simulink model "P3p3"  (R2017a)
settings: Solver=ode1  StartTime=0.0  StopTime=inf  FixedStep=0.01  RelTol=1e-3  EnableMultiTasking=on
PostLoadFcn:
  | qc_set_target_type(getConfigSet(bdroot, 'QUARC Default Target Configuration'));
values from neighbouring files (symbols this model uses):
  Joystick_gain_x = 1    [P3p3_init.m]
  Joystick_gain_y = -1    [P3p3_init.m]
  K = lqr(A_PI, B_PI, Q, R)    [P3p3_init.m]
  l_2 = g*(l_c*m_c - 2*m_p * l_h)    (= -0.659232)    [P3p3_init.m]
  l_3 = l_h * k_f    (= 0.10464)    [P3p3_init.m]
  P = inv(C_P*inv(B_P*K(:,1:3) - A_P) * B_P)    [P3p3_init.m]
undefined symbols (not defined in the file or in its folder): HIL, qc_get_step_size
libraries: simulink_extras x6, quarc_library x4
settings Model: SimulationMode=external  ExtModeTrigDuration=5000  Creator=Rchan  LastModifiedBy=Jakob
settings SolverCC: PositivePriorityOrder=on
settings DataIOCC: LimitDataPoints=on  SaveFormat=Array  SignalLoggingSaveFormat=ModelDataLogs
settings OptimizationCC: ExpressionDepthLimit=2147483647  InitFltsAndDblsToZero=on  LifeSpan=inf
settings DebuggingCC: SaveWithParameterizedLinksMsg=none  UnderspecifiedInitializationDetection=Classic  MergeDetectMultiDrivingBlocksExec=none  SolverPrmCheckMsg=warning  MultiTaskDSMMsg=warning  MultiTaskCondExecSysMsg=none  FcnCallInpInsideContextMsg=warning  StateNameClashWarn=warning  SFUnexpectedBacktrackingDiag=warning  SFNoUnconditionalDefaultTransitionDiag=warning  SFExecutionAtInitializationDiag=none
settings HardwareCC: ProdBitPerPointer=32  ProdBitPerSizeT=32  ProdBitPerPtrDiffT=32  ProdLargestAtomicFloat=None  ProdIntDivRoundTo=Undefined  ProdEndianess=Unspecified  ProdWordSize=32  ProdHWDeviceType=32-bit Generic
settings ModelReferenceCC: PropagateSignalLabelsOutOfModel=off
settings RTWCC: SystemTargetFile=quarc_win64.tlc  TemplateMakefile=quarc_default_tmf  Description=QUARC Win64 Target
settings STFCustomTargetCC: TargetPreCompLibLocation=C:\PROGRA~3\QUARC\lib\2014a\win64\release  ConcurrentExecutionCompliant=on  GeneratePreprocessorConditionals=Disable all  CPPClassGenCompliant=on  SystemTargetFile=quarc_win64.tlc
settings GRTTargetCC: TargetPreCompLibLocation=C:\PROGRA~3\QUARC\lib\2014a\win64\release  TargetLangStandard=C89/C90 (ANSI)  ParMdlRefBuildCompliant=off  CompOptLevelCompliant=off  GeneratePreprocessorConditionals=Disable all  CombineOutputUpdateFcns=off  MatFileLogging=off  GRTInterface=on  UseToolchainInfoCompliant=off  ExtMode=on  ExtModeMexFile=quarc_comm
settings ConfigComp: CovMetricSettings=dw  CovHtmlReporting=on  CovSaveCumulativeToWorkspaceVar=on  CovSaveSingleToWorkspaceVar=on  CovExternalEMLEnable=off  CovSFcnEnable=off

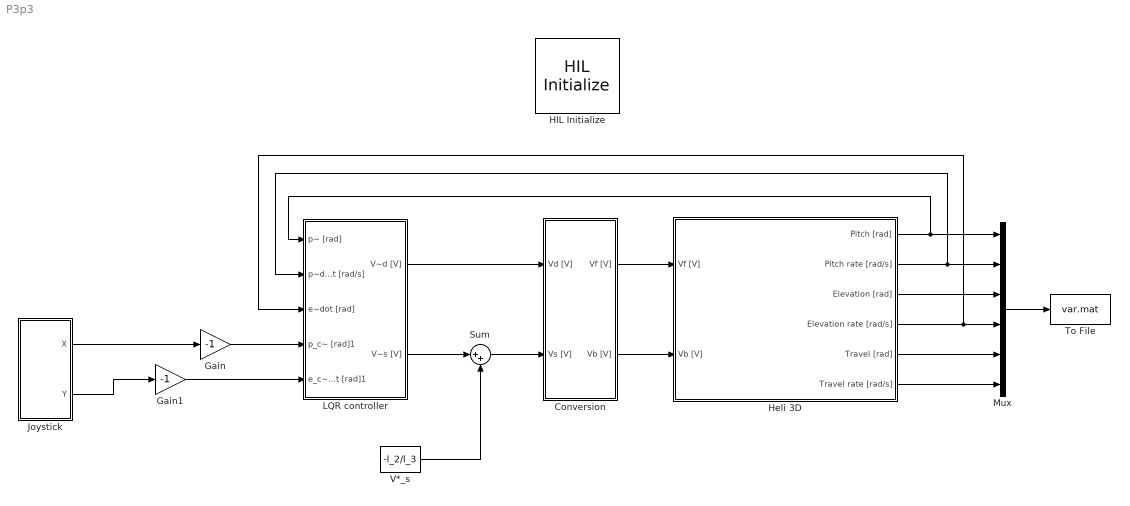
== system P3p3 ==
  Conversion : Subsystem
  Gain : Gain  Gain=-1
  Gain1 : Gain  Gain=-1
  HIL Initialize : quarc_library/Data Acquisition/Generic/Configuration/HIL Initialize  Priority=-99  object_name=HIL-1  board_type=q8_usb  board_number=0  board_options=update_rate=normal;decimation=1  exclusive=off  active=off  hardware_clocks=[0:2]  clock_modes=[]  initial_clock_frequencies=[]  set_clock_params_at_start=off  set_clock_params_at_switch_in=off  set_clock_frequencies_at_start=off  set_clock_frequencies_at_switch_in=off  analog_input_channels=[0:7]  analog_input_maximums=10  analog_input_minimums=-10  set_analog_input_params_at_start=on  set_analog_input_params_at_switch_in=off  analog_output_channels=[0:7]  analog_output_maximums=10  analog_output_minimums=-10  initial_analog_outputs=[0]  final_analog_outputs=[0]  watchdog_analog_outputs=0  set_analog_output_params_at_start=on  set_analog_output_params_at_switch_in=off  set_analog_outputs_at_start=on  set_analog_outputs_at_switch_in=off  set_analog_outputs_at_terminate=on  set_analog_outputs_at_switch_out=off  set_analog_outputs_on_watchdog=off  digital_input_channels=[]  digital_output_channels=[]  digital_output_configuration=[]  initial_digital_outputs=[1]  final_digital_outputs=[1]  watchdog_digital_outputs=[1]  set_digital_output_params_at_start=off  set_digital_output_params_at_switch_in=off  set_digital_outputs_at_start=on  set_digital_outputs_at_switch_in=off  set_digital_outputs_at_terminate=on  set_digital_outputs_at_switch_out=off  set_digital_outputs_on_watchdog=off  encoder_channels=[0:7]  quadrature=[4]  encoder_filter_frequency=[]  initial_encoder_counts=[0]  set_encoder_params_at_start=on  set_encoder_params_at_switch_in=off  set_encoder_counts_at_start=on  set_encoder_counts_at_switch_in=off  pwm_channels=[0:7]  pwm_modes=0  pwm_frequency=99.532799999999995e6/4095  pwm_configuration=[0]  pwm_alignment=[0]  pwm_polarity=[1]  pwm_leading_deadband=[0]  pwm_trailing_deadband=[0]  initial_pwm_outputs=[0]  final_pwm_outputs=[0]  watchdog_pwm_outputs=[0]  set_pwm_params_at_start=on  set_pwm_params_at_switch_in=off  set_pwm_outputs_at_start=on  set_pwm_outputs_at_switch_in=off  set_pwm_outputs_at_terminate=on  set_pwm_outputs_at_switch_out=off  set_pwm_outputs_on_watchdog=off  other_output_channels=[]  initial_other_outputs=[]  final_other_outputs=[]  watchdog_other_outputs=[]  set_other_outputs_at_start=off  set_other_outputs_at_switch_in=off  set_other_outputs_at_terminate=off  set_other_outputs_at_switch_out=off  set_other_outputs_on_watchdog=off
  Heli 3D : Subsystem
  Joystick : Subsystem
  LQR controller : Subsystem
  Mux : Mux  Inputs=6
  Sum : Sum  Inputs=|++
  To File : ToFile  Filename=var.mat  MatrixName=var
  V*_s : Constant  Value=-l_2/l_3
  wires:
  Conversion/2(Vb [V]) -> Heli 3D/2(Vb [V])
  Conversion/1(Vf [V]) -> Heli 3D/1(Vf [V])
  Heli 3D/5(Travel [rad]) -> Mux/5
  Heli 3D/6(Travel rate [rad/s]) -> Mux/6
  Heli 3D/1(Pitch [rad]) -> Mux/1, LQR controller/1(p~ [rad])
  Heli 3D/2(Pitch rate [rad/s]) -> Mux/2, LQR controller/2(p~dot [rad/s])
  Mux/1 -> To File/1
  Heli 3D/4(Elevation rate [rad/s]) -> LQR controller/3(e~dot [rad]), Mux/4
  Heli 3D/3(Elevation [rad]) -> Mux/3
  Joystick/1(X) -> Gain/1
  LQR controller/1("V~d [V] ") -> Conversion/1(Vd [V])
  Gain1/1 -> LQR controller/5(e_c~dot [rad]1)
  Gain/1 -> LQR controller/4(p_c~ [rad]1)
  Joystick/2(Y) -> Gain1/1
  V*_s/1 -> Sum/2
  Sum/1 -> Conversion/2(Vs [V])
  LQR controller/2(V~s [V]) -> Sum/1

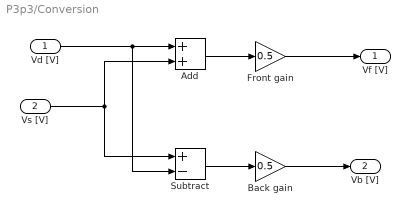
== system P3p3/Conversion ==
  Vd [V] : Inport
  Vs [V] : Inport  Port=2
  Add : Sum
  Back gain : Gain  Gain=0.5
  Front gain : Gain  Gain=0.5
  Subtract : Sum  Inputs=+-
  Vf [V] : Outport
  Vb [V] : Outport  Port=2
  wires:
  Vd [V]/1 -> Subtract/2, Add/1
  Vs [V]/1 -> Subtract/1, Add/2
  Subtract/1 -> Back gain/1
  Back gain/1 -> Vb [V]/1
  Add/1 -> Front gain/1
  Front gain/1 -> Vf [V]/1

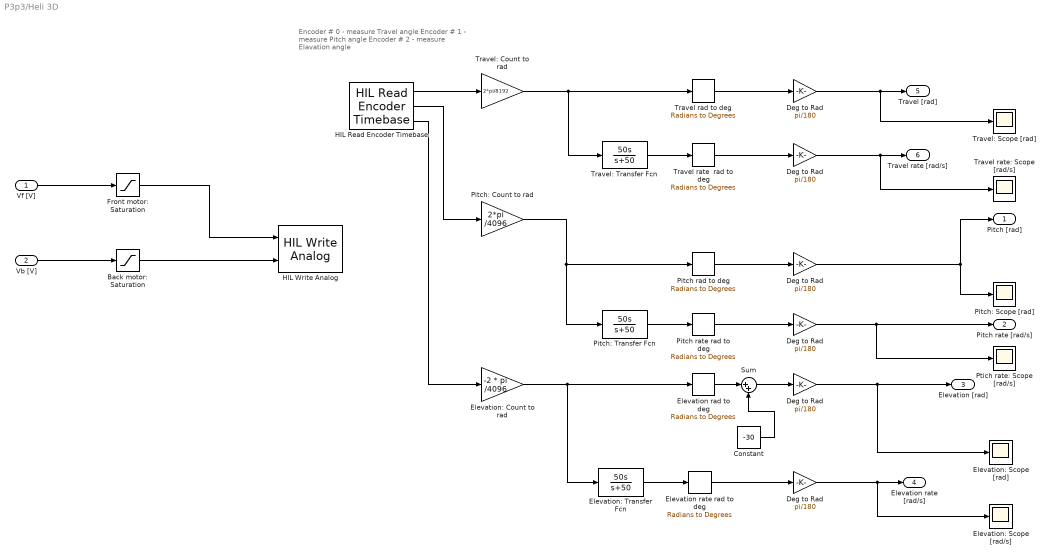
== system P3p3/Heli 3D ==
  note: Encoder # 0 - measure Travel angle
      | Encoder # 1 - measure Pitch angle
      | Encoder # 2 - measure Elavation angle
  Vf [V] : Inport
  Vb [V] : Inport  Port=2
  Back motor: Saturation : Saturate  UpperLimit=5  LowerLimit=-5
  Constant : Constant  Value=-30
  Deg to Rad : Gain  Gain=pi/180
  "Deg to Rad  " : Gain  Gain=pi/180
  "Deg to Rad   " : Gain  Gain=pi/180
  "Deg to Rad    " : Gain  Gain=pi/180
  "Deg to Rad     " : Gain  Gain=pi/180
  "Deg to Rad      " : Gain  Gain=pi/180
  Elevation rad to deg : simulink_extras/Transformations/Radians to Degrees
  Elevation rate rad to deg : simulink_extras/Transformations/Radians to Degrees
  Elevation: Count to rad : Gain  Gain=-2 * pi /4096
  Elevation: Scope [rad/s] : Scope
  Elevation: Scope [rad] : Scope
  Elevation: Transfer Fcn : TransferFcn  Numerator=[50 0]  Denominator=[1 50]
  Front motor: Saturation : Saturate  UpperLimit=5  LowerLimit=-5
  HIL Read Encoder Timebase : quarc_library/Data Acquisition/Generic/Timebases/HIL Read Encoder Timebase  object_name=HIL-1  clock=0  channels=[0:2]  samples_in_buffer=max(ceil(1/qc_get_step_size), 1)  active=on  vector_output=off  data_type_mode=Inherit via back propagation  data_type=double
  HIL Write Analog : quarc_library/Data Acquisition/Generic/Immediate I//O/HIL Write Analog  object_name=HIL-1  channels=[0:1]  sample_time=-1  active=off  vector_input=off
  Pitch rad to deg : simulink_extras/Transformations/Radians to Degrees
  Pitch rate rad to deg : simulink_extras/Transformations/Radians to Degrees
  Pitch: Count to rad : Gain  Gain=2*pi /4096
  Pitch: Scope [rad] : Scope
  Pitch: Transfer Fcn : TransferFcn  Numerator=[50 0]  Denominator=[1 50]
  Ptich rate: Scope [rad/s] : Scope
  Sum : Sum  Inputs=|++
  Travel rad to deg : simulink_extras/Transformations/Radians to Degrees
  Travel rate  rad to deg : simulink_extras/Transformations/Radians to Degrees
  Travel rate: Scope [rad/s] : Scope
  Travel: Count to rad : Gain  Gain=2*pi/8192
  Travel: Scope [rad] : Scope
  Travel: Transfer Fcn : TransferFcn  Numerator=[50 0]  Denominator=[1 50]
  Pitch [rad] : Outport
  Pitch rate [rad/s] : Outport  Port=2
  Elevation [rad] : Outport  Port=3
  Elevation rate [rad/s] : Outport  Port=4
  Travel [rad] : Outport  Port=5
  Travel rate [rad/s] : Outport  Port=6
  wires:
  HIL Read Encoder Timebase/1 -> Travel: Count to rad/1
  HIL Read Encoder Timebase/2 -> Pitch: Count to rad/1
  HIL Read Encoder Timebase/3 -> Elevation: Count to rad/1
  Travel: Count to rad/1 -> Travel: Transfer Fcn/1, Travel rad to deg/1
  Travel: Transfer Fcn/1 -> Travel rate  rad to deg/1
  Pitch: Count to rad/1 -> Pitch: Transfer Fcn/1, Pitch rad to deg/1
  Pitch: Transfer Fcn/1 -> Pitch rate rad to deg/1
  Elevation: Count to rad/1 -> Elevation: Transfer Fcn/1, Elevation rad to deg/1
  Elevation: Transfer Fcn/1 -> Elevation rate rad to deg/1
  Travel rad to deg/1 -> Deg to Rad/1
  Travel rate  rad to deg/1 -> "Deg to Rad  "/1
  Pitch rate rad to deg/1 -> "Deg to Rad    "/1
  Elevation rate rad to deg/1 -> "Deg to Rad      "/1
  Vf [V]/1 -> Front motor: Saturation/1
  Vb [V]/1 -> Back motor: Saturation/1
  Front motor: Saturation/1 -> HIL Write Analog/1
  Back motor: Saturation/1 -> HIL Write Analog/2
  Pitch rad to deg/1 -> "Deg to Rad   "/1
  Constant/1 -> Sum/2
  Sum/1 -> "Deg to Rad     "/1
  Elevation rad to deg/1 -> Sum/1
  "Deg to Rad  "/1 -> Travel rate: Scope [rad/s]/1, Travel rate [rad/s]/1
  Deg to Rad/1 -> Travel: Scope [rad]/1, Travel [rad]/1
  "Deg to Rad   "/1 -> Pitch [rad]/1, Pitch: Scope [rad]/1
  "Deg to Rad    "/1 -> Ptich rate: Scope [rad/s]/1, Pitch rate [rad/s]/1
  "Deg to Rad     "/1 -> Elevation: Scope [rad]/1, Elevation [rad]/1
  "Deg to Rad      "/1 -> Elevation: Scope [rad/s]/1, Elevation rate [rad/s]/1

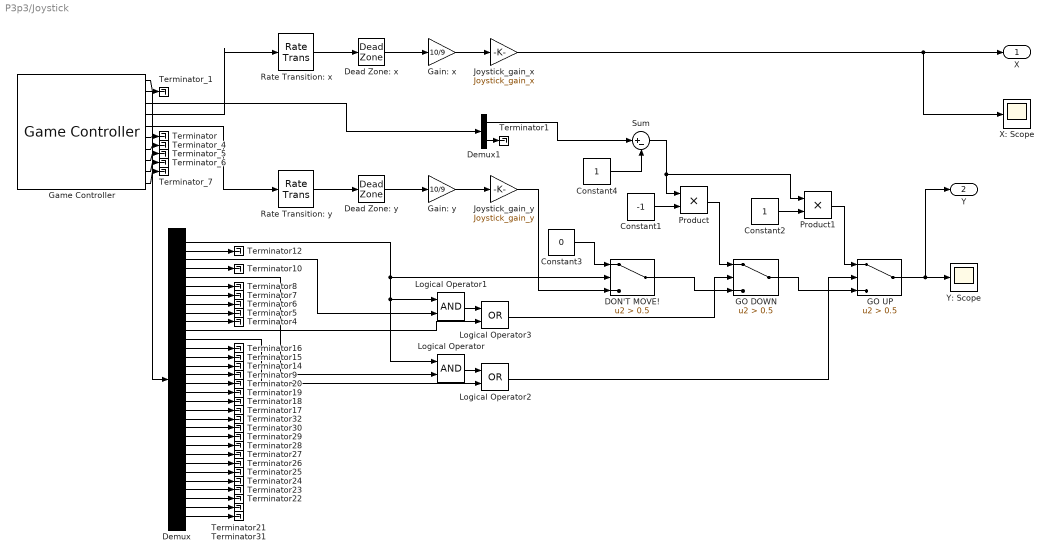
== system P3p3/Joystick ==
  Constant1 : Constant  Value=-1  SampleTime=-1
  Constant2 : Constant  SampleTime=-1
  Constant3 : Constant  Value=0  SampleTime=-1
  Constant4 : Constant  SampleTime=-1
  DON'T MOVE! : Switch  Criteria=u2 > Threshold  Threshold=0.5
  Dead Zone: x : DeadZone  LowerValue=-0.1  UpperValue=0.1  SaturateOnIntegerOverflow=on
  Dead Zone: y : DeadZone  LowerValue=-0.1  UpperValue=0.1  SaturateOnIntegerOverflow=on
  Demux : Demux  Outputs=32
  Demux1 : Demux  Outputs=2
  GO DOWN : Switch  Criteria=u2 > Threshold  Threshold=0.5
  GO UP : Switch  Criteria=u2 > Threshold  Threshold=0.5
  Gain: x : Gain  Gain=10/9
  Gain: y : Gain  Gain=10/9
  Game Controller : quarc_library/Devices/Peripherals/Target/Game Controller  controller=1  buffer_size=12  deadzone=[]  saturation=[]  sample_time=max(qc_get_step_size, 0.01)  auto_center=off  enabled=on
  Joystick_gain_x : Gain  Gain=Joystick_gain_x
  Joystick_gain_y : Gain  Gain=Joystick_gain_y
  Logical Operator : Logic  AllPortsSameDT=off  OutDataTypeStr=boolean
  Logical Operator1 : Logic  AllPortsSameDT=off  OutDataTypeStr=boolean
  Logical Operator2 : Logic  Operator=OR  AllPortsSameDT=off  OutDataTypeStr=boolean
  Logical Operator3 : Logic  Operator=OR  AllPortsSameDT=off  OutDataTypeStr=boolean
  Product : Product
  Product1 : Product
  Rate Transition: x : RateTransition
  Rate Transition: y : RateTransition
  Sum : Sum  Inputs=|+-
  Terminator{,1,4..10,12,14..32} (29 alike) : Terminator
  Terminator_{1,4..7} (5 alike) : Terminator
  X: Scope : Scope
  Y: Scope : Scope
  X : Outport
  Y : Outport  Port=2
  wires:
  Rate Transition: y/1 -> Dead Zone: y/1
  Rate Transition: x/1 -> Dead Zone: x/1
  Game Controller/5 -> Rate Transition: y/1
  Game Controller/4 -> Rate Transition: x/1
  Game Controller/1 -> Terminator_1/1
  Game Controller/7 -> Terminator_4/1
  Game Controller/8 -> Terminator_5/1
  Game Controller/9 -> Terminator_6/1
  Game Controller/10 -> Terminator_7/1
  Game Controller/3 -> Demux1/1
  Game Controller/6 -> Terminator/1
  Dead Zone: x/1 -> Gain: x/1
  Dead Zone: y/1 -> Gain: y/1
  Gain: x/1 -> Joystick_gain_x/1
  Gain: y/1 -> Joystick_gain_y/1
  Game Controller/2 -> Demux/1
  Demux/2 -> Terminator12/1
  Demux/4 -> Terminator10/1
  Demux/7 -> Terminator7/1
  Demux/8 -> Terminator6/1
  Demux/9 -> Terminator5/1
  Demux/10 -> Terminator4/1
  Demux/11 -> Logical Operator3/2
  Demux/12 -> Logical Operator2/2
  Demux/14 -> Terminator15/1
  Demux/15 -> Terminator14/1
  Demux/16 -> Terminator9/1
  Demux/13 -> Terminator16/1
  Demux/17 -> Terminator20/1
  Demux/18 -> Terminator19/1
  Demux/19 -> Terminator18/1
  Demux/20 -> Terminator17/1
  Demux/22 -> Terminator30/1
  Demux/23 -> Terminator29/1
  Demux/24 -> Terminator28/1
  Demux/25 -> Terminator27/1
  Demux/26 -> Terminator26/1
  Demux/27 -> Terminator25/1
  Demux/28 -> Terminator24/1
  Demux/30 -> Terminator22/1
  Demux/31 -> Terminator21/1
  Demux/32 -> Terminator31/1
  Demux/29 -> Terminator23/1
  Demux/21 -> Terminator32/1
  Joystick_gain_x/1 -> X: Scope/1, X/1
  GO DOWN/1 -> GO UP/3
  GO UP/1 -> Y/1, Y: Scope/1
  Constant3/1 -> DON'T MOVE!/1
  Joystick_gain_y/1 -> DON'T MOVE!/3
  Demux/1 -> Logical Operator1/1, Logical Operator/1, DON'T MOVE!/2
  DON'T MOVE!/1 -> GO DOWN/3
  Demux/6 -> Terminator8/1
  Demux/3 -> Logical Operator1/2
  Demux/5 -> Logical Operator/2
  Logical Operator/1 -> Logical Operator2/1
  Logical Operator3/1 -> GO DOWN/2
  Logical Operator1/1 -> Logical Operator3/1
  Logical Operator2/1 -> GO UP/2
  Demux1/2 -> Terminator1/1
  Constant1/1 -> Product/2
  Constant2/1 -> Product1/2
  Product/1 -> GO DOWN/1
  Product1/1 -> GO UP/1
  Demux1/1 -> Sum/1
  Sum/1 -> Product1/1, Product/1
  Constant4/1 -> Sum/2

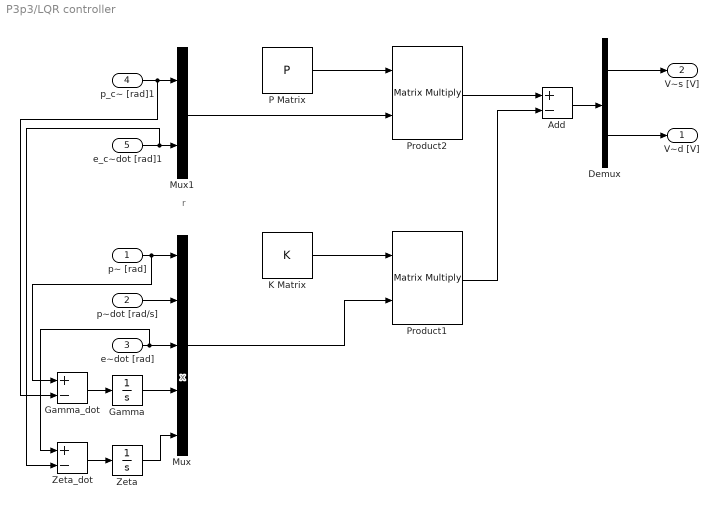
== system P3p3/LQR controller ==
  note: x
  note: r
  p~ [rad] : Inport
  p~dot [rad/s] : Inport  Port=2
  e~dot [rad] : Inport  Port=3
  p_c~ [rad]1 : Inport  Port=4
  e_c~dot [rad]1 : Inport  Port=5
  Add : Sum  Inputs=+-
  Demux : Demux  Outputs=2
  Gamma : Integrator
  Gamma_dot : Sum  Inputs=+-
  K Matrix : Constant  Value=K
  Mux : Mux  Inputs=5
  Mux1 : Mux  Inputs=2
  P Matrix : Constant  Value=P
  Product1 : Product  Multiplication=Matrix(*)
  Product2 : Product  Multiplication=Matrix(*)
  Zeta : Integrator
  Zeta_dot : Sum  Inputs=+-
  "V~d [V] " : Outport  InitialOutput=0
  V~s [V] : Outport  Port=2  InitialOutput=0
  wires:
  p~dot [rad/s]/1 -> Mux/2
  e~dot [rad]/1 -> Zeta_dot/1, Mux/3
  p_c~ [rad]1/1 -> Gamma_dot/2, Mux1/1
  e_c~dot [rad]1/1 -> Zeta_dot/2, Mux1/2
  Mux/1 -> Product1/2
  K Matrix/1 -> Product1/1
  Mux1/1 -> Product2/2
  P Matrix/1 -> Product2/1
  Product1/1 -> Add/2
  Product2/1 -> Add/1
  Add/1 -> Demux/1
  Demux/1 -> V~s [V]/1
  Demux/2 -> "V~d [V] "/1
  p~ [rad]/1 -> Gamma_dot/1, Mux/1
  Zeta/1 -> Mux/5
  Gamma_dot/1 -> Gamma/1
  Gamma/1 -> Mux/4
  Zeta_dot/1 -> Zeta/1
